simulink model "test_model_pas"  (R2019b)
settings: Solver=VariableStepAuto  StartTime=0.0  StopTime=2  RelTol=1e-3
values from neighbouring files (symbols this model uses):
  dq0 = [0; 0; 8]    [run_simulation.m]    (also in test_simulink.m)
  q0 = [pi/9; -pi/9; 0]    [run_simulation.m]    (also in test_simulink.m)
  x0 = [q0;dq0]    [test_simulink.m]
libraries: dspinverses x1
settings Model: Creator=Niilouf  LastModifiedBy=Niilouf

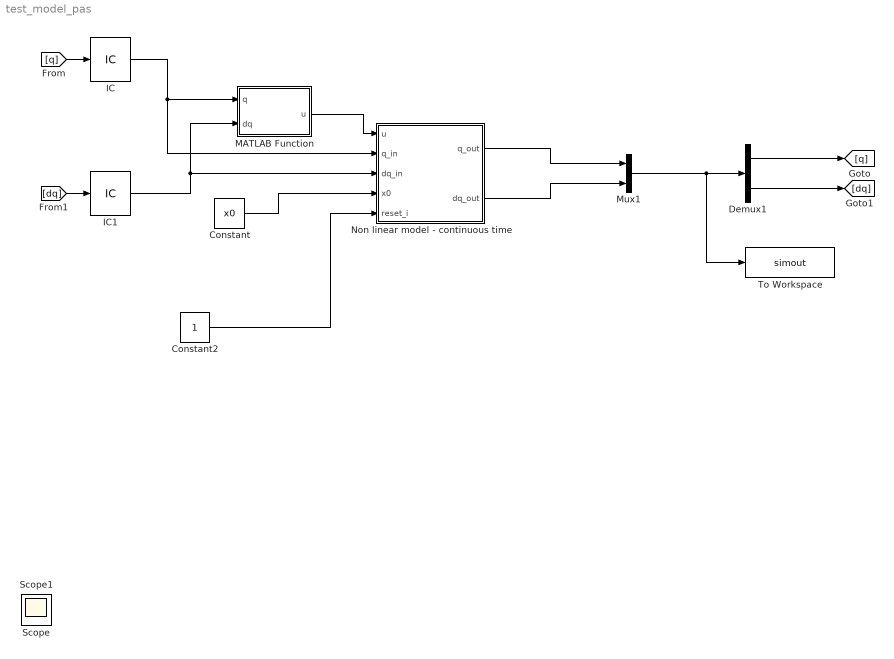
== system test_model_pas ==
  Constant : Constant  Value=x0
  Constant2 : Constant
  Demux1 : Demux  Outputs=2
  IC : InitialCondition  Value=q0
  IC1 : InitialCondition  Value=dq0
  MATLAB Function : MATLAB Function  TreatAsAtomicUnit=on
  Mux1 : Mux  Inputs=2
  Non linear model - continuous time : Subsystem
  To Workspace : ToWorkspace  VariableName=simout  SaveFormat=Timeseries  SampleTime=-1
  Scope : Scope
  Scope1 : Scope
  wires:
  Demux1/1 -> [q]
  Demux1/2 -> [dq]
  [q] -> IC/1
  [dq] -> IC1/1
  IC/1 -> MATLAB Function/1(q), Non linear model - continuous time/2(q_in)
  IC1/1 -> MATLAB Function/2(dq), Non linear model - continuous time/3(dq_in)
  ? -> ?
  MATLAB Function/1(u) -> Non linear model - continuous time/1(u)
  Constant/1 -> Non linear model - continuous time/4(x0)
  Constant2/1 -> Non linear model - continuous time/5("reset_i ")
  Non linear model - continuous time/2(dq_out) -> Mux1/2
  Non linear model - continuous time/1(q_out) -> Mux1/1
  Mux1/1 -> To Workspace/1, Demux1/1

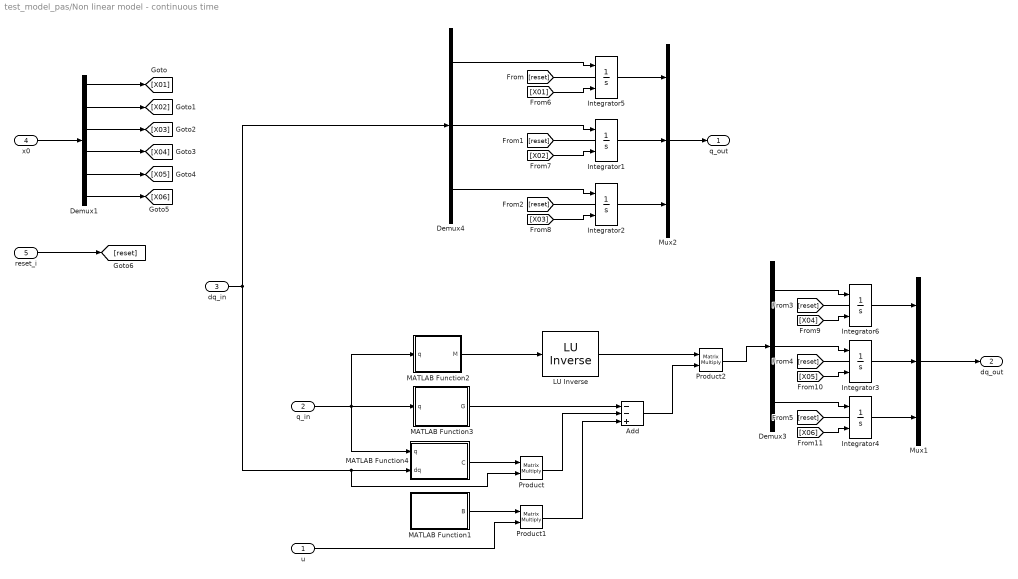
== system test_model_pas/Non linear model - continuous time ==
  u : Inport  PortDimensions=2
  q_in : Inport  Port=2  PortDimensions=3
  dq_in : Inport  Port=3  PortDimensions=3
  x0 : Inport  Port=4  PortDimensions=6
  "reset_i " : Inport  Port=5
  " LU Inverse" : dspinverses/ LU Inverse
      settings: SourceProductName=DSP System Toolbox
  Add : Sum  Inputs=--+
  Demux1 : Demux  Outputs=6
  Demux3 : Demux  Outputs=3
  Demux4 : Demux  Outputs=3
  Integrator{1..6} (6 alike) : Integrator  InitialConditionSource=external  InitialCondition=x0(1)
  MATLAB Function1 : MATLAB Function  TreatAsAtomicUnit=on
  MATLAB Function2 : MATLAB Function  TreatAsAtomicUnit=on
  MATLAB Function3 : MATLAB Function  TreatAsAtomicUnit=on
  MATLAB Function4 : MATLAB Function  TreatAsAtomicUnit=on
  Mux1 : Mux  Inputs=3
  Mux2 : Mux  Inputs=3
  Product : Product  Multiplication=Matrix(*)
  Product1 : Product  Multiplication=Matrix(*)
  Product2 : Product  Multiplication=Matrix(*)
  q_out : Outport  PortDimensions=3  VectorParamsAs1DForOutWhenUnconnected=off
  dq_out : Outport  Port=2  PortDimensions=3  VectorParamsAs1DForOutWhenUnconnected=off
  wires:
  Demux4/1 -> Integrator5/1
  q_in/1 -> MATLAB Function2/1(q), MATLAB Function4/1(q), MATLAB Function3/1(q)
  Mux2/1 -> q_out/1
  dq_in/1 -> Demux4/1, MATLAB Function4/2(dq), Product/2
  Mux1/1 -> dq_out/1
  MATLAB Function4/1(C) -> Product/1
  MATLAB Function1/1(B) -> Product1/1
  MATLAB Function3/1(G) -> Add/1
  Product1/1 -> Add/3
  Product/1 -> Add/2
  Add/1 -> Product2/2
  Product2/1 -> Demux3/1
  MATLAB Function2/1(M) -> " LU Inverse"/1
  " LU Inverse"/1 -> Product2/1
  u/1 -> Product1/2
  Demux4/2 -> Integrator1/1
  Demux4/3 -> Integrator2/1
  x0/1 -> Demux1/1
  Demux3/1 -> Integrator6/1
  Integrator6/1 -> Mux1/1
  Integrator3/1 -> Mux1/2
  Integrator4/1 -> Mux1/3
  Demux3/2 -> Integrator3/1
  Demux3/3 -> Integrator4/1
  Integrator5/1 -> Mux2/1
  Integrator1/1 -> Mux2/2
  Integrator2/1 -> Mux2/3
  Demux1/1 -> [X01]
  Demux1/2 -> [X02]
  Demux1/3 -> [X03]
  Demux1/4 -> [X04]
  Demux1/5 -> [X05]
  Demux1/6 -> [X06]
  "reset_i "/1 -> [reset]
  [reset] -> ?
  [reset] -> ?
  [reset] -> ?
  [X01] -> Integrator5/2
  [X03] -> Integrator2/2
  [X02] -> Integrator1/2
  [reset] -> ?
  [X04] -> Integrator6/2
  [reset] -> ?
  [reset] -> ?
  [X05] -> Integrator3/2
  [X06] -> Integrator4/2

== matlab function test_model_pas/MATLAB Function ==
  data: u output; q input; dq input
function u = control(q, dq)
% You may call control_hyper_parameters and desired_outputs in this function
% you don't necessarily need to use all the inputs to this control function

% extract parameters
kp1 = 457.5;
kp2 = 161;
kd1 = 77.05; 
kd2 = 5;
alpha = 10.4 * pi / 180;

% controller for torso
u1 = kp1*q(3)-alpha + kd1*dq(3);

% controller for legs
u2 = -kp2*(q(2)+q(1)) - kd2*(dq(2)+dq(1));

% saturate the output torque
u = [u1; u2];
u = max(min(u, 30), -30); 

end

== matlab function test_model_pas/Non linear model - continuous time/MATLAB Function1 ==
  data: B output
function B = eval_B()
%EVAL_B
%    B = EVAL_B

%    This function was generated by the Symbolic Math Toolbox version 7.1.
%    14-Oct-2018 18:44:49

B = reshape([1.0,0.0,-1.0,0.0,1.0,-1.0],[3,2]);
end

== matlab function test_model_pas/Non linear model - continuous time/MATLAB Function2 ==
  data: M output; q input
function M = eval_M(q)
%EVAL_M
%    M = EVAL_M(L1,L2,L3,M1,M2,M3,Q1,Q2,Q3)

%    This function was generated by the Symbolic Math Toolbox version 7.1.
%    14-Oct-2018 18:44:47
q1 = q(1);
q2 = q(2);
q3 = q(3);

[m1, m2, m3, l1, l2, l3, ~] = set_parameters();

t2 = q1-q2;
t3 = cos(t2);
t4 = q1-q3;
t5 = cos(t4);
t6 = l1.*l3.*m3.*t5.*(1.0./2.0);
M = reshape([l1.^2.*(m1.*(1.0./4.0)+m2+m3),l1.*l2.*m2.*t3.*(-1.0./2.0),t6,l1.*l2.*m2.*t3.*(-1.0./2.0),l2.^2.*m2.*(1.0./4.0),0.0,t6,0.0,l3.^2.*m3.*(1.0./4.0)],[3,3]);

== matlab function test_model_pas/Non linear model - continuous time/MATLAB Function3 ==
  data: G output; q input
function G = eval_G(q)
%EVAL_G
%    G = EVAL_G(G,L1,L2,L3,M1,M2,M3,Q1,Q2,Q3)

%    This function was generated by the Symbolic Math Toolbox version 7.1.
%    14-Oct-2018 18:44:49
q1 = q(1);
q2 = q(2);
q3 = q(3);

[m1, m2, m3, l1, l2, l3, g] = set_parameters();

G = [g.*l1.*sin(q1).*(m1+m2.*2.0+m3.*2.0).*(-1.0./2.0);g.*l2.*m2.*sin(q2).*(1.0./2.0);g.*l3.*m3.*sin(q3).*(-1.0./2.0)];

== matlab function test_model_pas/Non linear model - continuous time/MATLAB Function4 ==
  data: C output; q input; dq input
function C = eval_C(q, dq)
%EVAL_C
%    C = EVAL_C(DQ1,DQ2,DQ3,L1,L2,L3,M2,M3,Q1,Q2,Q3)

%    This function was generated by the Symbolic Math Toolbox version 7.1.
%    14-Oct-2018 18:44:48

q1 = q(1);
q2 = q(2);
q3 = q(3);
dq1 = dq(1);
dq2 = dq(2);
dq3 = dq(3);

[m1, m2, m3, l1, l2, l3, ~] = set_parameters();

t2 = q1-q2;
t3 = sin(t2);
t4 = q1-q3;
t5 = sin(t4);
C = reshape([0.0,dq1.*l1.*l2.*m2.*t3.*(1.0./2.0),dq1.*l1.*l3.*m3.*t5.*(-1.0./2.0),dq2.*l1.*l2.*m2.*t3.*(-1.0./2.0),0.0,0.0,dq3.*l1.*l3.*m3.*t5.*(1.0./2.0),0.0,0.0],[3,3]);
end
